simulink subsystem "SCDynamics_FreeTorque"  (R2021a)
settings: Solver=VariableStepAuto  StartTime=0.0  StopTime=10.0  RelTol=1e-3
undefined symbols (not defined in the file): Ix, Iy, Iz, mu, q0, r0, v0, w0
libraries: aerolibutil x1
settings Model: Creator=Laura  LastModifiedBy=Laura

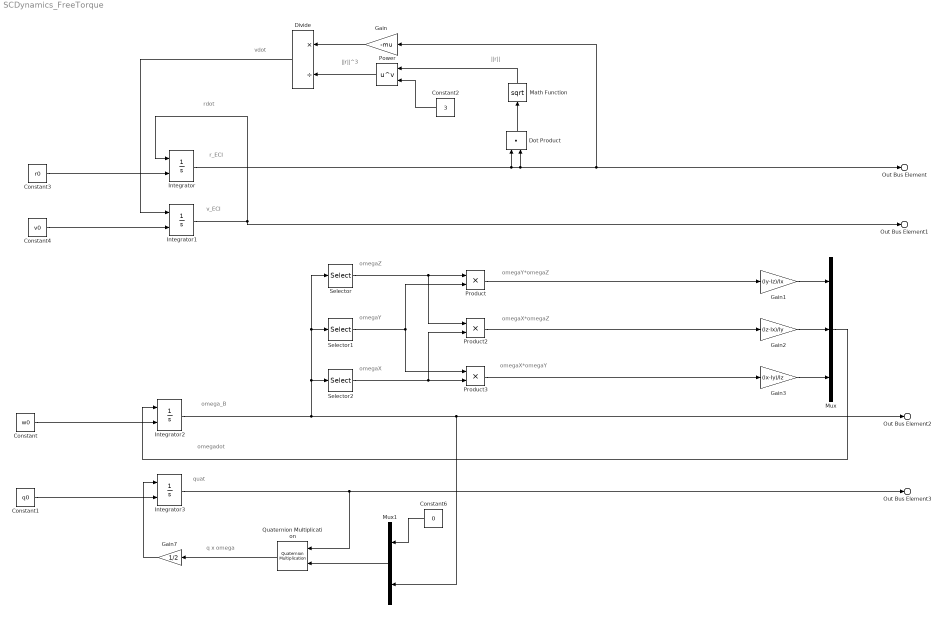
== system SCDynamics_FreeTorque ==
  note: rdot
  note: r_ECI
  note: vdot
  note: omegadot
  note: omegaX
  note: omegaY
  note: omega_B
  note: ||r||
  note: ||r||^3
  note: v_ECI
  note: omegaX*omegaY
  note: quat
  note: omegaZ
  note: q x omega
  note: omegaY*omegaZ
  note: omegaX*omegaZ
  Constant : Constant  Value=w0
  Constant1 : Constant  Value=q0
  Constant2 : Constant  Value=3
  Constant3 : Constant  Value=r0
  Constant4 : Constant  Value=v0
  Constant6 : Constant  Value=0
  Divide : Product  Inputs=*/
  Dot Product : DotProduct  InputSameDT=on  OutDataTypeStr=Inherit: Inherit via internal rule
  Gain : Gain  Gain=-mu
  Gain1 : Gain  Gain=(Iy-Iz)/Ix
  Gain2 : Gain  Gain=(Iz-Ix)/Iy
  Gain3 : Gain  Gain=(Ix-Iy)/Iz
  Gain7 : Gain  Gain=1/2
  Integrator{,1..3} (4 alike) : Integrator  InitialConditionSource=external
  Math Function : Math  Operator=sqrt  SignedPower=on  SaturateOnIntegerOverflow=on
  Mux : Mux  Inputs=3
  Mux1 : Mux  Inputs=2
  Power : Math  Operator=pow  SaturateOnIntegerOverflow=on
  Product : Product
  Product2 : Product
  Product3 : Product
  Quaternion Multiplication : aerolibutil/Quaternion Multiplication
  Selector : Selector  InputPortWidth=3  IndexOptions=Index vector (dialog)  Indices=[3]  OutputSizes=1
  Selector1 : Selector  InputPortWidth=3  IndexOptions=Index vector (dialog)  Indices=[2]  OutputSizes=1
  Selector2 : Selector  InputPortWidth=3  IndexOptions=Index vector (dialog)  Indices=[1]  OutputSizes=1
  Out Bus Element : Outport  PortName=DynamicsOut  Element=r_ECI
  Out Bus Element1 : Outport  PortName=DynamicsOut  Element=v_ECI
  Out Bus Element2 : Outport  PortName=DynamicsOut  Element=omega_B
  Out Bus Element3 : Outport  PortName=DynamicsOut  Element=quat
  wires:
  Gain3/1 -> Mux/3
  Constant1/1 -> Integrator3/2
  Math Function/1 -> Power/1
  Divide/1 -> Integrator1/1
  Gain7/1 -> Integrator3/1
  Constant/1 -> Integrator2/2
  Product/1 -> Gain1/1
  Power/1 -> Divide/2
  Selector/1 -> Product2/1, Product/1
  Product2/1 -> Gain2/1
  Constant4/1 -> Integrator1/2
  Product3/1 -> Gain3/1
  Selector1/1 -> Product/2, Product3/1
  Mux1/1 -> Quaternion Multiplication/2
  Integrator/1 -> Gain/1, Out Bus Element/1, Dot Product/2, Dot Product/1
  Gain2/1 -> Mux/2
  Integrator3/1 -> Quaternion Multiplication/1, Out Bus Element3/1
  Quaternion Multiplication/1 -> Gain7/1
  Dot Product/1 -> Math Function/1
  Gain/1 -> Divide/1
  Constant6/1 -> Mux1/1
  Integrator1/1 -> Integrator/1, Out Bus Element1/1
  Mux/1 -> Integrator2/1
  Gain1/1 -> Mux/1
  Integrator2/1 -> Selector2/1, Selector1/1, Selector/1, Mux1/2, Out Bus Element2/1
  Constant2/1 -> Power/2
  Constant3/1 -> Integrator/2
  Selector2/1 -> Product2/2, Product3/2
